simulink model "Droop_GC"  (Simulink 9.1)
settings: Solver=ode4  StartTime=0.0  StopTime=2.6  FixedStep=1e-6  RelTol=1e-3  EnableMultiTasking=on
InitFcn:
  | %% Circuit parameters
  | % LC filter
  | Lf_1 = 1.35e-3;
  | Rf_1 = 0.1;
  | Cf_1 = 50e-6;
  | 
  | Lf_2 = 1.35e-3;
  | Rf_2 = 0.1;
  | Cf_2 = 50e-6;
  | 
  | Lf_3 = 1.35e-3;
  | Rf_3 = 0.1;
  | Cf_3 = 50e-6;
  | 
  | % transmission line(grid coupling impedance)
  | L_1 = 0.35e-3;
  | R_1 = 0.03;
  | 
  | L_2 = 0.35e-3;
  | R_2 = 0.03;
  | 
  | L_3 = 0.35e-3;
  | R_3 = 0.03;
  | 
  | % Network
  | % active power loop
  | fn = 50;
  | wn = 2*pi*fn;
  | 
  | R_line_1 = 0.23;
  | L_line_1 = 0.1 / wn;
  | 
  | R_line_2 = 0.35;
  | L_line_2 = 0.58 / wn;
  | 
  | 
  | %% Control parameters
  | % power measurement LPF
  | wc = 31.41;
  | 
  | % Power droop
  | mp_1 = mp;
  | mp_2 = mp;
  | mp_3 = mp;
  | 
  | nq_1 = nq;
  | nq_2 = nq;
  | nq_3 = nq;
  | 
  | J1 = 0.1;
  | J2 = 0.1;
  | J3 = 0.1;
  | 
  | Pref_1 = Pref;
  | Pref_2 = Pref;
  | Pref_3 = Pref;
  | 
  | % outer voltage loop
  | Kpv_1 = 0.05;
  | Kiv_1 = 390;
  | F_1 = 1;
  | 
  | Kpv_2 = 0.05;
  | Kiv_2 = 390;
  | F_2 = 1;
  | 
  | Kpv_3 = 0.05;
  | Kiv_3 = 390;
  | F_3 = 1;
  | 
  | % inner current control loop
  | Kpc_1 = 10.5;
  | Kic_1 = 16e3;
  | 
  | Kpc_2 = 10.5;
  | Kic_2 = 16e3;
  | 
  | Kpc_3 = 10.5;
  | Kic_3 = 16e3;
  | % ?? reference voltage
  | 
  | V_phase_rms = 220;
  | V_line_rms = V_phase_rms * sqrt(3);
  | 
  | % Load
  | R_load_1 = R1;
  | L_load_1 = 10e-9;
  | 
  | R_load_2 = R3;
  | L_load_2 = 10e-9;
  | 
  | 
  | % Pre Synchronisation for Con 1
  | t_grid_breaker = 0.6;
  | t_preSyn_start = 0.01;
  | t_preSyn_end = t_grid_breaker;
  | 
  | % Pre Synchronisation for Con 2
  | t_grid_breaker_2 = 1.2;
  | t_preSyn_start_2 = 0.61;
  | t_preSyn_end_2 = t_grid_breaker_2;
  | 
  | 
  | % Pre Synchronisation for Con 3
  | t_grid_breaker_3 = 1.8;
  | t_preSyn_start_3 = 1.21;
  | t_preSyn_end_3 = t_grid_breaker_3;
  | 
  | % PLL
  | Vg = V_phase_rms * sqrt(2);
  | % Disturbance Rejection
  | wd = 2*pi*100;                      % Definition of 1st Harmonic Band
  | att_lim = 20*log10((5e-3)/108);      % Defintion of Damping here: 5e-3 maximum tolerance and 108 V Type E negative sequence Voltage
  | 
  | a = 2.4;                            % corresponds xi = 0.7
  | 
  | wc_lim = wd*sqrt(Vg)/sqrt(a)*10^(att_lim/40);    % calculation of bandwidth
  | 
  | Kp_pll = wc_lim;
  | wf_pll = a*wc_lim;      %1/sqrt(2)*w0;
  | T_L = 1/wf_pll;
  | Ki_pll = Kp_pll*wc_lim/a;
  | Ti_pll = Kp_pll/Ki_pll;
  | 
  | %% Pre synchronization PI parameters? G_cl =(Kp_syn*s + Ki_syn) / (s^2 + Kp_syn*s + Ki_syn)
  | % ? = 0.707? ts = ??
  | ts_syn = 0.5;
  | zeta_syn = 0.707;
  | wn_syn = 4.5 / (ts_syn * zeta_syn);
  | 
  | Ki_syn = wn_syn * wn_syn;
  | Kp_syn = 2 * zeta_syn * wn_syn;
  | 
  | 
  | Udc = 800;
  | fs = 8000;
values from neighbouring files (symbols this model uses):
  mp = 9.4e-5    (= 9.4e-05)    [model_coefficient.m]
  nq = 1.3e-3    (= 0.0013)    [model_coefficient.m]
  Pref = 10000    [model_coefficient.m]
  R1 = 25    [model_coefficient.m]
  R3 = 20    [model_coefficient.m]
libraries: powerlib x53, powerlib_meascontrol x25
(part 1 of 2)
Description:
  | Model of a simple control system for use iin training.
settings Model: ARTEMISmethode_block_infos=$$__separator__$$Droop_GC/ARTEMIS Guide$$__separator__$$  Creator=Paul Baracos  LastModifiedBy=10135
settings DataIOCC: LimitDataPoints=on  SignalLoggingSaveFormat=ModelDataLogs  SaveOutput=off  SaveTime=off  ReturnWorkspaceOutputs=on  SignalLoggingName=sigsOut  LoggingIntervals=[2.599, 2.6]
settings OptimizationCC: BlockReduction=off  BooleanDataType=off  OptimizeBlockIOStorage=off  BufferReuse=off  GlobalBufferReuse=off  ExpressionFolding=off  LocalBlockOutputs=off  InitFltsAndDblsToZero=on  OptimizeDataStoreBuffers=off  BusAssignmentInplaceUpdate=off
settings DebuggingCC: SaveWithParameterizedLinksMsg=none  SignalResolutionControl=TryResolveAllWithWarning  MultiTaskDSMMsg=warning  MultiTaskCondExecSysMsg=none  FcnCallInpInsideContextMsg=warning
settings HardwareCC: TargetUnknown=on
settings GRTTargetCC: TargetFcnLib=ansi_tfl_tmw.mat  GeneratePreprocessorConditionals=Disable all
settings SimscapeCC: SimscapeNormalizeSystem=off  SimscapeLogType=local  SimscapeLogLimitData=off

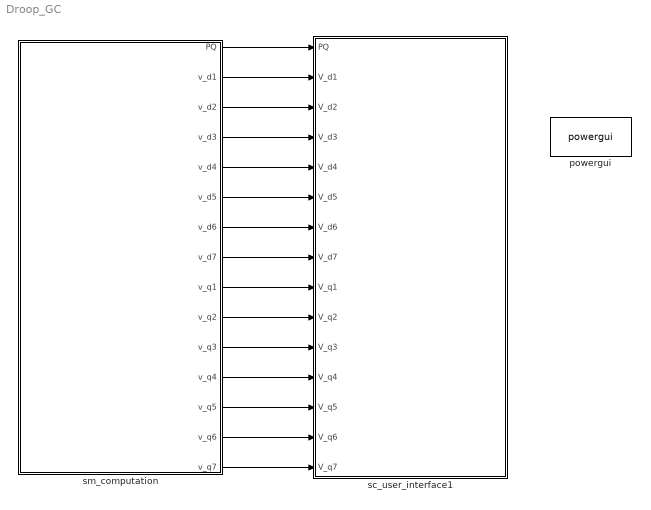
== system Droop_GC ==
  powergui : powerlib/powergui  Priority=1  SimulationMode=Discrete  SampleTime=1e-6  frequency=60  Iterations=50  frequencyindice=0  Pbase=100e6  ErrMax=1e-4  UnitsV=kV  UnitsW=MW  buscounter=0  FunctionMessages=off  echomessages=off  EnableUseOfTLC=off  CurrentSourceSwitches=off  DisableSnubberDevices=off  DisableRonSwitches=off  DisableVfSwitches=off  DisplayEquations=off  SolverType=Tustin/Backward Euler (TBE)  Interpol=off  ExternalGateDelay=off  methode=off  Ts=100  x0status=blocks  SPID=off  SwTol=0  HookPort=off  RestoreLinks=warning  ResistiveCurrentMeasurement=off  Frange=[0:2:500]  Ylog=off  Xlog=on  ShowGrid=off  save=off  variable=ZData  structure=0  ZoomFFT=off  StartTime=0.0  cycles=1  DisplayStyle=1  fundamental=60  FreqAxis=off  MaxFrequency=1000  frequencyindicesteady=1  RmsSteady=1  display=off
  sc_user_interface1 : Subsystem
  sm_computation : Subsystem
  wires:
  sm_computation/1(PQ) -> sc_user_interface1/1(PQ)
  sm_computation/2(v_d1) -> sc_user_interface1/2(V_d1)
  sm_computation/3(v_d2) -> sc_user_interface1/3(V_d2)
  sm_computation/4(v_d3) -> sc_user_interface1/4(V_d3)
  sm_computation/5(v_d4) -> sc_user_interface1/5(V_d4)
  sm_computation/6(v_d5) -> sc_user_interface1/6(V_d5)
  sm_computation/7(v_d6) -> sc_user_interface1/7(V_d6)
  sm_computation/8(v_d7) -> sc_user_interface1/8(V_d7)
  sm_computation/9(v_q1) -> sc_user_interface1/9(V_q1)
  sm_computation/10(v_q2) -> sc_user_interface1/10(V_q2)
  sm_computation/11(v_q3) -> sc_user_interface1/11(V_q3)
  sm_computation/12(v_q4) -> sc_user_interface1/12(V_q4)
  sm_computation/13(v_q5) -> sc_user_interface1/13(V_q5)
  sm_computation/14(v_q6) -> sc_user_interface1/14(V_q6)
  sm_computation/15(v_q7) -> sc_user_interface1/15(V_q7)

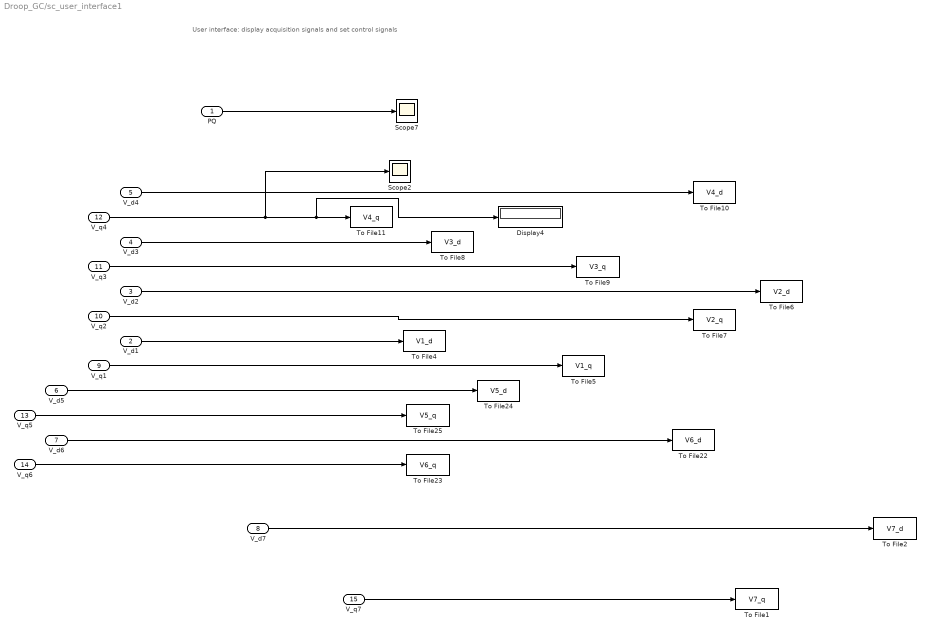
== system Droop_GC/sc_user_interface1 ==
  note: User interface: display acquisition signals and set control signals
  PQ : Inport
  V_d1 : Inport  Port=2
  V_d2 : Inport  Port=3
  V_d3 : Inport  Port=4
  V_d4 : Inport  Port=5
  V_d5 : Inport  Port=6
  V_d6 : Inport  Port=7
  V_d7 : Inport  Port=8
  V_q1 : Inport  Port=9
  V_q2 : Inport  Port=10
  V_q3 : Inport  Port=11
  V_q4 : Inport  Port=12
  V_q5 : Inport  Port=13
  V_q6 : Inport  Port=14
  V_q7 : Inport  Port=15
  Display4 : Display
  Scope2 : Scope
      settings: Tag=op_tm_save_it
  Scope7 : Scope
      settings: Tag=op_tm_save_it
  To File1 : ToFile  Filename=V7_q  SaveFormat=Timeseries
  To File10 : ToFile  Filename=V4_d  SaveFormat=Timeseries
  To File11 : ToFile  Filename=V4_q  SaveFormat=Timeseries
  To File2 : ToFile  Filename=V7_d  SaveFormat=Timeseries
  To File22 : ToFile  Filename=V6_d  SaveFormat=Timeseries
  To File23 : ToFile  Filename=V6_q  SaveFormat=Timeseries
  To File24 : ToFile  Filename=V5_d  SaveFormat=Timeseries
  To File25 : ToFile  Filename=V5_q  SaveFormat=Timeseries
  To File4 : ToFile  Filename=V1_d  SaveFormat=Timeseries
  To File5 : ToFile  Filename=V1_q  SaveFormat=Timeseries
  To File6 : ToFile  Filename=V2_d  SaveFormat=Timeseries
  To File7 : ToFile  Filename=V2_q  SaveFormat=Timeseries
  To File8 : ToFile  Filename=V3_d  SaveFormat=Timeseries
  To File9 : ToFile  Filename=V3_q  SaveFormat=Timeseries
  wires:
  PQ/1 -> Scope7/1
  V_d6/1 -> To File22/1
  V_d2/1 -> To File6/1
  V_q3/1 -> To File9/1
  V_q2/1 -> To File7/1
  V_q5/1 -> To File25/1
  V_d5/1 -> To File24/1
  V_d3/1 -> To File8/1
  V_q6/1 -> To File23/1
  V_d1/1 -> To File4/1
  V_q1/1 -> To File5/1
  V_q4/1 -> Scope2/1, Display4/1, To File11/1
  V_d4/1 -> To File10/1
  V_q7/1 -> To File1/1
  V_d7/1 -> To File2/1

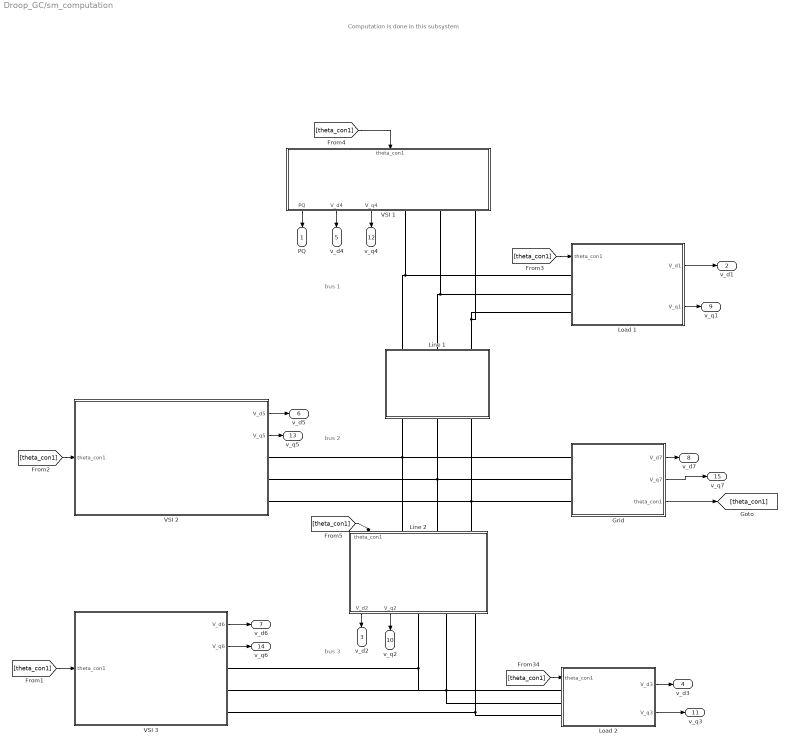
== system Droop_GC/sm_computation ==
  note: Computation is done in this subsystem
  note: bus 1
  note: bus 3
  note: bus 2
  Grid : Subsystem
  Line 1 : Subsystem
  Line 2 : Subsystem
  Load 1 : Subsystem
  Load 2 : Subsystem
  VSI 1 : Subsystem
  VSI 2 : Subsystem
  VSI 3 : Subsystem
  PQ : Outport
  v_d1 : Outport  Port=2
  v_d2 : Outport  Port=3
  v_d3 : Outport  Port=4
  v_d4 : Outport  Port=5
  v_d5 : Outport  Port=6
  v_d6 : Outport  Port=7
  v_d7 : Outport  Port=8
  v_q1 : Outport  Port=9
  v_q2 : Outport  Port=10
  v_q3 : Outport  Port=11
  v_q4 : Outport  Port=12
  v_q5 : Outport  Port=13
  v_q6 : Outport  Port=14
  v_q7 : Outport  Port=15
  wires:
  Grid/3(theta_con1) -> [theta_con1]
  [theta_con1] -> Load 2/1("theta_con1 ")
  [theta_con1] -> VSI 3/1("theta_con1 ")
  [theta_con1] -> VSI 2/1("theta_con1 ")
  [theta_con1] -> Load 1/1("theta_con1 ")
  [theta_con1] -> VSI 1/1("theta_con1 ")
  VSI 1/1(PQ) -> PQ/1
  Load 1/1(V_d1) -> v_d1/1
  Line 2/1(V_d2) -> v_d2/1
  Load 2/1(V_d3) -> v_d3/1
  VSI 1/2(V_d4) -> v_d4/1
  VSI 2/1(V_d5) -> v_d5/1
  VSI 3/1(V_d6) -> v_d6/1
  Grid/1(V_d7) -> v_d7/1
  Load 1/2(V_q1) -> v_q1/1
  Line 2/2(V_q2) -> v_q2/1
  Load 2/2(V_q3) -> v_q3/1
  VSI 1/3(V_q4) -> v_q4/1
  VSI 2/2(V_q5) -> v_q5/1
  VSI 3/2(V_q6) -> v_q6/1
  Grid/2(V_q7) -> v_q7/1
  [theta_con1] -> Line 2/1("theta_con1 ")
  connections:
  Load 2/LConn1 -- VSI 3/RConn1 -- Line 2/RConn1
  VSI 1/RConn1 -- Load 1/LConn1 -- Line 1/LConn1
  VSI 1/RConn3 -- Line 1/LConn3 -- Load 1/LConn3
  Grid/LConn1 -- Line 2/LConn1 -- VSI 2/RConn1 -- Line 1/RConn1
  Grid/LConn3 -- Line 2/LConn3 -- VSI 2/RConn3 -- Line 1/RConn3
  Load 2/LConn2 -- VSI 3/RConn2 -- Line 2/RConn2
  VSI 1/RConn2 -- Line 1/LConn2 -- Load 1/LConn2
  Grid/LConn2 -- Line 2/LConn2 -- VSI 2/RConn2 -- Line 1/RConn2
  Load 2/LConn3 -- VSI 3/RConn3 -- Line 2/RConn3

== system Droop_GC/sm_computation/Grid ==
  Constant1 : Constant  Value=2*pi/3
  Constant3 : Constant  Value=wn
  Demux : Demux  Outputs=3
  Demux1 : Demux  Outputs=3
  Gain : Gain  Gain=Vg
  Integrator3 : Integrator
  Mux : Mux  Inputs=3
  Sum : Sum  Inputs=|+-
  Sum1 : Sum  Inputs=++|
  Terminator2 : Terminator
  Three-Phase Series RLC Branch : powerlib/Elements/Three-Phase Series RLC Branch  LConnTagsString=A|B|C  RConnTagsString=A|B|C  BranchType=RL  Resistance=R_line_1  Inductance=L_line_1  Capacitance=1e-6  Measurements=None
  Three-Phase V-I Measurement : powerlib/Measurements/Three-Phase V-I Measurement  VoltageMeasurement=phase-to-ground  SetLabelV=off  LabelV=Vabc  Vpu=off  VpuLL=off  CurrentMeasurement=no  SetLabelI=off  LabelI=Iabc  Ipu=off  Pbase=100e6  Vbase=500e3  OutputType=Complex  PhasorSimulation=off  PSBequivalent=0
  Trigonometric Function : Trigonometry  Operator=cos
  Trigonometric Function1 : Trigonometry  Operator=cos
  Trigonometric Function2 : Trigonometry  Operator=cos
  abc to dq0 : powerlib_meascontrol/Transformations/abc to dq0  Alignment=Aligned with phase A axis
  u1 : powerlib/Electrical Sources/Controlled Voltage Source  Initialize=off  Source_Type=AC  Amplitude=0  Phase=0  Frequency=50  Measurements=None
  u2 : powerlib/Electrical Sources/Controlled Voltage Source  Initialize=off  Source_Type=AC  Amplitude=0  Phase=0  Frequency=50  Measurements=None
  u3 : powerlib/Electrical Sources/Controlled Voltage Source  Initialize=off  Source_Type=AC  Amplitude=0  Phase=0  Frequency=50  Measurements=None
  A : PMIOPort  Side=Left
  B : PMIOPort  Port=2  Side=Left
  C : PMIOPort  Port=3  Side=Left
  V_d7 : Outport
  V_q7 : Outport  Port=2
  theta_con1 : Outport  Port=3
  tag scope: theta_con1=global
  wires:
  Constant3/1 -> Integrator3/1
  Integrator3/1 -> Trigonometric Function/1, Sum1/2, Sum/1, theta_con1/1, [theta_con1]
  Demux/2 -> u2/1
  Demux/1 -> u1/1
  Demux/3 -> u3/1
  Constant1/1 -> Sum1/1, Sum/2
  Sum1/1 -> Trigonometric Function2/1
  Sum/1 -> Trigonometric Function1/1
  Trigonometric Function/1 -> Mux/1
  Trigonometric Function2/1 -> Mux/3
  Trigonometric Function1/1 -> Mux/2
  Mux/1 -> Gain/1
  Gain/1 -> Demux/1
  Demux1/2 -> V_q7/1
  abc to dq0/1 -> Demux1/1
  Three-Phase V-I Measurement/1 -> abc to dq0/1
  [theta_con1] -> abc to dq0/2
  Demux1/3 -> Terminator2/1
  Demux1/1 -> V_d7/1
  connections:
  Three-Phase V-I Measurement/RConn2 -- u2/RConn1
  Three-Phase V-I Measurement/RConn1 -- u1/RConn1
  Three-Phase V-I Measurement/RConn3 -- u3/RConn1
  Three-Phase Series RLC Branch/RConn1 -- Three-Phase V-I Measurement/LConn1
  Three-Phase Series RLC Branch/RConn2 -- Three-Phase V-I Measurement/LConn2
  Three-Phase Series RLC Branch/RConn3 -- Three-Phase V-I Measurement/LConn3
  Three-Phase Series RLC Branch/LConn1 -- A/RConn1
  Three-Phase Series RLC Branch/LConn2 -- B/RConn1
  Three-Phase Series RLC Branch/LConn3 -- C/RConn1
  u1/LConn1 -- u3/LConn1 -- u2/LConn1

== system Droop_GC/sm_computation/Line 1 ==
  Three-Phase Series RLC Branch : powerlib/Elements/Three-Phase Series RLC Branch  LConnTagsString=A|B|C  RConnTagsString=A|B|C  BranchType=RL  Resistance=R_line_1  Inductance=L_line_1  Capacitance=1e-6  Measurements=None
  Three-Phase V-I Measurement : powerlib/Measurements/Three-Phase V-I Measurement  VoltageMeasurement=phase-to-ground  SetLabelV=off  LabelV=Vabc  Vpu=off  VpuLL=off  CurrentMeasurement=yes  SetLabelI=off  LabelI=Iabc  Ipu=off  Pbase=100e6  Vbase=500e3  OutputType=Complex  PhasorSimulation=off  PSBequivalent=0
  a : PMIOPort  Side=Right
  b : PMIOPort  Port=2  Side=Right
  c : PMIOPort  Port=3  Side=Right
  A1 : PMIOPort  Port=4  Side=Left
  B1 : PMIOPort  Port=5  Side=Left
  C1 : PMIOPort  Port=6  Side=Left
  tag scope: I_line_1_abc=global, V_b_1_abc=global
  wires:
  Three-Phase V-I Measurement/1 -> [V_b_1_abc]
  Three-Phase V-I Measurement/2 -> [I_line_1_abc]
  connections:
  Three-Phase Series RLC Branch/RConn1 -- a/RConn1
  Three-Phase Series RLC Branch/RConn2 -- b/RConn1
  Three-Phase Series RLC Branch/RConn3 -- c/RConn1
  Three-Phase Series RLC Branch/LConn2 -- Three-Phase V-I Measurement/RConn2
  C1/RConn1 -- Three-Phase V-I Measurement/LConn3
  B1/RConn1 -- Three-Phase V-I Measurement/LConn2
  Three-Phase Series RLC Branch/LConn3 -- Three-Phase V-I Measurement/RConn3
  A1/RConn1 -- Three-Phase V-I Measurement/LConn1
  Three-Phase Series RLC Branch/LConn1 -- Three-Phase V-I Measurement/RConn1

== system Droop_GC/sm_computation/Line 2 ==
  "theta_con1 " : Inport
  Demux : Demux  Outputs=3
  Terminator2 : Terminator
  Three-Phase Series RLC Branch : powerlib/Elements/Three-Phase Series RLC Branch  LConnTagsString=A|B|C  RConnTagsString=A|B|C  BranchType=RL  Resistance=R_line_2  Inductance=L_line_2  Capacitance=1e-6  Measurements=None
  Three-Phase V-I Measurement : powerlib/Measurements/Three-Phase V-I Measurement  VoltageMeasurement=phase-to-ground  SetLabelV=off  LabelV=Vabc  Vpu=off  VpuLL=off  CurrentMeasurement=no  SetLabelI=off  LabelI=Iabc  Ipu=off  Pbase=100e6  Vbase=500e3  OutputType=Complex  PhasorSimulation=off  PSBequivalent=0
  Three-Phase V-I Measurement1 : powerlib/Measurements/Three-Phase V-I Measurement  VoltageMeasurement=no  SetLabelV=off  LabelV=Vabc  Vpu=off  VpuLL=off  CurrentMeasurement=no  SetLabelI=off  LabelI=Iabc  Ipu=off  Pbase=100e6  Vbase=500e3  OutputType=Complex  PhasorSimulation=off  PSBequivalent=0
  abc to dq0 : powerlib_meascontrol/Transformations/abc to dq0  Alignment=Aligned with phase A axis
  a : PMIOPort  Side=Right
  b : PMIOPort  Port=2  Side=Right
  c : PMIOPort  Port=3  Side=Right
  A1 : PMIOPort  Port=4  Side=Left
  B1 : PMIOPort  Port=5  Side=Left
  C1 : PMIOPort  Port=6  Side=Left
  V_d2 : Outport
  V_q2 : Outport  Port=2
  wires:
  Demux/3 -> Terminator2/1
  Demux/2 -> V_q2/1
  Three-Phase V-I Measurement/1 -> abc to dq0/1
  "theta_con1 "/1 -> abc to dq0/2
  abc to dq0/1 -> Demux/1
  Demux/1 -> V_d2/1
  connections:
  B1/RConn1 -- Three-Phase V-I Measurement/LConn2
  Three-Phase Series RLC Branch/LConn2 -- Three-Phase V-I Measurement/RConn2
  Three-Phase V-I Measurement/RConn1 -- Three-Phase Series RLC Branch/LConn1
  Three-Phase V-I Measurement/RConn3 -- Three-Phase Series RLC Branch/LConn3
  A1/RConn1 -- Three-Phase V-I Measurement/LConn1
  C1/RConn1 -- Three-Phase V-I Measurement/LConn3
  Three-Phase Series RLC Branch/RConn1 -- Three-Phase V-I Measurement1/LConn1
  Three-Phase Series RLC Branch/RConn2 -- Three-Phase V-I Measurement1/LConn2
  Three-Phase Series RLC Branch/RConn3 -- Three-Phase V-I Measurement1/LConn3
  c/RConn1 -- Three-Phase V-I Measurement1/RConn3
  b/RConn1 -- Three-Phase V-I Measurement1/RConn2
  a/RConn1 -- Three-Phase V-I Measurement1/RConn1

== system Droop_GC/sm_computation/Load 1 ==
  "theta_con1 " : Inport
  Demux : Demux  Outputs=3
  Ground2 : powerlib/Elements/Ground  LConnTagsString=a
  Terminator2 : Terminator
  Three-Phase Series RLC Branch : powerlib/Elements/Three-Phase Series RLC Branch  LConnTagsString=A|B|C  RConnTagsString=A|B|C  BranchType=RL  Resistance=R_load_1  Inductance=L_load_1  Capacitance=1e-6  Measurements=None
  Three-Phase V-I Measurement : powerlib/Measurements/Three-Phase V-I Measurement  VoltageMeasurement=phase-to-ground  SetLabelV=off  LabelV=Vabc  Vpu=off  VpuLL=off  CurrentMeasurement=no  SetLabelI=off  LabelI=Iabc  Ipu=off  Pbase=100e6  Vbase=500e3  OutputType=Complex  PhasorSimulation=off  PSBequivalent=0
  abc to dq0 : powerlib_meascontrol/Transformations/abc to dq0  Alignment=Aligned with phase A axis
  A : PMIOPort  Side=Left
  B : PMIOPort  Port=2  Side=Left
  C : PMIOPort  Port=3  Side=Left
  V_d1 : Outport
  V_q1 : Outport  Port=2
  wires:
  abc to dq0/1 -> Demux/1
  Three-Phase V-I Measurement/1 -> abc to dq0/1
  Demux/2 -> V_q1/1
  Demux/3 -> Terminator2/1
  Demux/1 -> V_d1/1
  "theta_con1 "/1 -> abc to dq0/2
  connections:
  Ground2/LConn1 -- Three-Phase Series RLC Branch/RConn3 -- Three-Phase Series RLC Branch/RConn1 -- Three-Phase Series RLC Branch/RConn2
  Three-Phase V-I Measurement/RConn2 -- Three-Phase Series RLC Branch/LConn2
  Three-Phase V-I Measurement/RConn1 -- Three-Phase Series RLC Branch/LConn1
  Three-Phase V-I Measurement/RConn3 -- Three-Phase Series RLC Branch/LConn3
  A/RConn1 -- Three-Phase V-I Measurement/LConn1
  B/RConn1 -- Three-Phase V-I Measurement/LConn2
  C/RConn1 -- Three-Phase V-I Measurement/LConn3

== system Droop_GC/sm_computation/Load 2 ==
  "theta_con1 " : Inport
  Demux : Demux  Outputs=3
  Ground2 : powerlib/Elements/Ground  LConnTagsString=a
  Terminator2 : Terminator
  Three-Phase Series RLC Branch : powerlib/Elements/Three-Phase Series RLC Branch  LConnTagsString=A|B|C  RConnTagsString=A|B|C  BranchType=RL  Resistance=R_load_2  Inductance=L_load_2  Capacitance=1e-6  Measurements=None
  Three-Phase V-I Measurement : powerlib/Measurements/Three-Phase V-I Measurement  VoltageMeasurement=phase-to-ground  SetLabelV=off  LabelV=Vabc  Vpu=off  VpuLL=off  CurrentMeasurement=no  SetLabelI=off  LabelI=Iabc  Ipu=off  Pbase=100e6  Vbase=500e3  OutputType=Complex  PhasorSimulation=off  PSBequivalent=0
  abc to dq0 : powerlib_meascontrol/Transformations/abc to dq0  Alignment=Aligned with phase A axis
  A : PMIOPort  Side=Left
  B : PMIOPort  Port=2  Side=Left
  C : PMIOPort  Port=3  Side=Left
  V_d3 : Outport
  V_q3 : Outport  Port=2
  wires:
  Demux/2 -> V_q3/1
  abc to dq0/1 -> Demux/1
  Three-Phase V-I Measurement/1 -> abc to dq0/1
  "theta_con1 "/1 -> abc to dq0/2
  Demux/3 -> Terminator2/1
  Demux/1 -> V_d3/1
  connections:
  Three-Phase Series RLC Branch/RConn1 -- Ground2/LConn1 -- Three-Phase Series RLC Branch/RConn3 -- Three-Phase Series RLC Branch/RConn2
  Three-Phase Series RLC Branch/LConn2 -- Three-Phase V-I Measurement/RConn2
  C/RConn1 -- Three-Phase V-I Measurement/LConn3
  B/RConn1 -- Three-Phase V-I Measurement/LConn2
  Three-Phase V-I Measurement/RConn3 -- Three-Phase Series RLC Branch/LConn3
  A/RConn1 -- Three-Phase V-I Measurement/LConn1
  Three-Phase V-I Measurement/RConn1 -- Three-Phase Series RLC Branch/LConn1

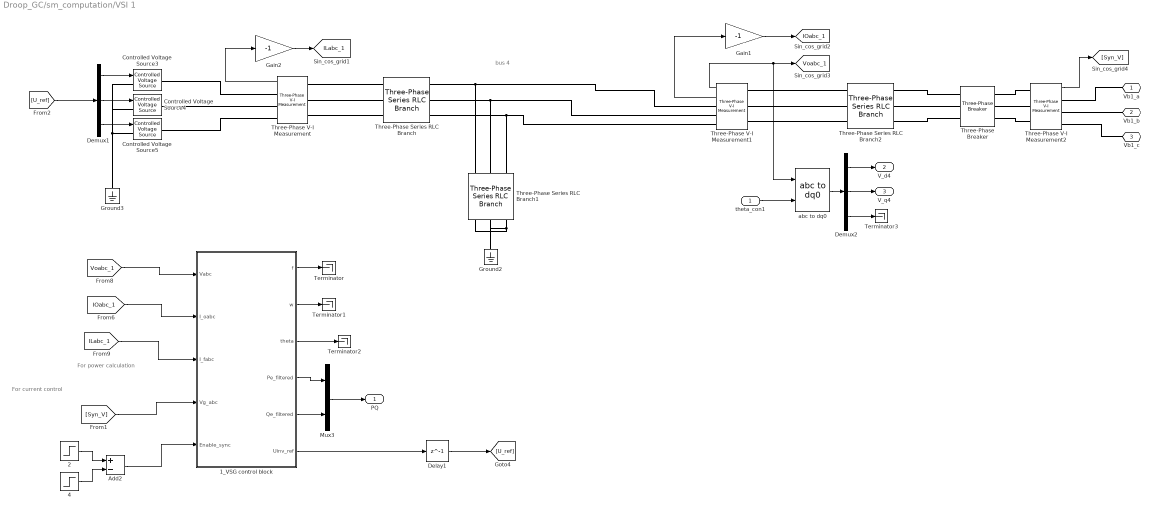
== system Droop_GC/sm_computation/VSI 1 ==
  note: For power calculation
  note: For current control
  note: bus 4
  "theta_con1 " : Inport
  " 2" : Step  Time=t_preSyn_start  SampleTime=0
  " 4" : Step  Time=t_preSyn_end  SampleTime=0
  1_VSG control block : Subsystem
  Add2 : Sum  Inputs=+-
  Controlled Voltage Source3 : powerlib/Electrical Sources/Controlled Voltage Source  Initialize=on  Source_Type=AC  Amplitude=0  Phase=0  Frequency=0  Measurements=None
  Controlled Voltage Source4 : powerlib/Electrical Sources/Controlled Voltage Source  Initialize=on  Source_Type=AC  Amplitude=0  Phase=0  Frequency=0  Measurements=None
  Controlled Voltage Source5 : powerlib/Electrical Sources/Controlled Voltage Source  Initialize=on  Source_Type=AC  Amplitude=0  Phase=0  Frequency=0  Measurements=None
  Delay1 : Delay  DelayLength=1  InitialCondition=0
  Demux1 : Demux  Outputs=3
  Demux2 : Demux  Outputs=3
  Gain1 : Gain  Gain=-1
  Gain2 : Gain  Gain=-1
  Ground2 : powerlib/Elements/Ground  LConnTagsString=a
  Ground3 : powerlib/Elements/Ground  LConnTagsString=a
  Mux3 : Mux  Inputs=2
  Terminator{,1..3} (4 alike) : Terminator
  Three-Phase Series RLC Branch : powerlib/Elements/Three-Phase Series RLC Branch  LConnTagsString=A|B|C  RConnTagsString=A|B|C  BranchType=RL  Resistance=Rf_1  Inductance=Lf_1  Capacitance=1e-6  Measurements=None
  Three-Phase Series RLC Branch1 : powerlib/Elements/Three-Phase Series RLC Branch  LConnTagsString=A|B|C  RConnTagsString=A|B|C  BranchType=C  Resistance=Rf_1  Inductance=0.1e-3  Capacitance=Cf_1  Measurements=None
  Three-Phase Series RLC Branch2 : powerlib/Elements/Three-Phase Series RLC Branch  LConnTagsString=A|B|C  RConnTagsString=A|B|C  BranchType=RL  Resistance=R_1  Inductance=L_1  Capacitance=1e-6  Measurements=None
  Three-Phase V-I Measurement : powerlib/Measurements/Three-Phase V-I Measurement  VoltageMeasurement=no  SetLabelV=off  LabelV=Vabc  Vpu=off  VpuLL=off  CurrentMeasurement=yes  SetLabelI=off  LabelI=Iabc  Ipu=off  Pbase=100e6  Vbase=500e3  OutputType=Complex  PhasorSimulation=off  PSBequivalent=0
  Three-Phase V-I Measurement1 : powerlib/Measurements/Three-Phase V-I Measurement  VoltageMeasurement=phase-to-ground  SetLabelV=off  LabelV=Vabc  Vpu=off  VpuLL=off  CurrentMeasurement=yes  SetLabelI=off  LabelI=Iabc  Ipu=off  Pbase=100e6  Vbase=500e3  OutputType=Complex  PhasorSimulation=off  PSBequivalent=0
  Three-Phase V-I Measurement2 : powerlib/Measurements/Three-Phase V-I Measurement  VoltageMeasurement=phase-to-ground  SetLabelV=off  LabelV=Vabc  Vpu=off  VpuLL=off  CurrentMeasurement=no  SetLabelI=off  LabelI=Iabc  Ipu=off  Pbase=100e6  Vbase=500e3  OutputType=Complex  PhasorSimulation=off  PSBequivalent=0
  Three-Phase Breaker : powerlib/Elements/Three-Phase Breaker  InitialState=open  SwitchA=on  SwitchB=on  SwitchC=on  SwitchTimes="[t_grid_breaker  20]"  External=off  BreakerResistance=0.00001  SnubberResistance=1e8  SnubberCapacitance=inf  Measurements=None
  abc to dq0 : powerlib_meascontrol/Transformations/abc to dq0  Alignment=Aligned with phase A axis
  Vb1_a : PMIOPort  Side=Right
  Vb1_b : PMIOPort  Port=2  Side=Right
  Vb1_c : PMIOPort  Port=3  Side=Right
  PQ : Outport
  V_d4 : Outport  Port=2
  V_q4 : Outport  Port=3
  tag scope: ILabc_1=global, IOabc_1=global, Voabc_1=global
  wires:
  [ILabc_1] -> 1_VSG control block/3(I_fabc)
  [Voabc_1] -> 1_VSG control block/1(Vabc)
  [IOabc_1] -> 1_VSG control block/2(I_oabc)
  Mux3/1 -> PQ/1
  1_VSG control block/4(Pe_filtered) -> Mux3/1
  1_VSG control block/5(Qe_filtered) -> Mux3/2
  1_VSG control block/2(w) -> Terminator1/1
  1_VSG control block/1(f) -> Terminator/1
  Three-Phase V-I Measurement2/1 -> [Syn_V]
  [Syn_V] -> 1_VSG control block/4(Vg_abc)
  " 2"/1 -> Add2/1
  " 4"/1 -> Add2/2
  Add2/1 -> 1_VSG control block/5(Enable_sync)
  1_VSG control block/3(theta) -> Terminator2/1
  Three-Phase V-I Measurement/1 -> Gain2/1
  Gain1/1 -> [IOabc_1]
  Three-Phase V-I Measurement1/2 -> Gain1/1
  Three-Phase V-I Measurement1/1 -> abc to dq0/1, [Voabc_1]
  Gain2/1 -> [ILabc_1]
  1_VSG control block/6(Uinv_ref) -> Delay1/1
  Delay1/1 -> [U_ref]
  [U_ref] -> Demux1/1
  Demux1/3 -> Controlled Voltage Source5/1
  Demux1/1 -> Controlled Voltage Source3/1
  Demux1/2 -> Controlled Voltage Source4/1
  Demux2/1 -> V_d4/1
  Demux2/2 -> V_q4/1
  Demux2/3 -> Terminator3/1
  abc to dq0/1 -> Demux2/1
  "theta_con1 "/1 -> abc to dq0/2
  connections:
  Three-Phase Series RLC Branch2/RConn2 -- Three-Phase Breaker/LConn2
  Three-Phase Series RLC Branch2/RConn1 -- Three-Phase Breaker/LConn1
  Three-Phase Series RLC Branch2/RConn3 -- Three-Phase Breaker/LConn3
  Three-Phase V-I Measurement2/LConn2 -- Three-Phase Breaker/RConn2
  Three-Phase Breaker/RConn1 -- Three-Phase V-I Measurement2/LConn1
  Three-Phase Breaker/RConn3 -- Three-Phase V-I Measurement2/LConn3
  Three-Phase V-I Measurement2/RConn1 -- Vb1_a/RConn1
  Three-Phase V-I Measurement2/RConn2 -- Vb1_b/RConn1
  Three-Phase V-I Measurement2/RConn3 -- Vb1_c/RConn1
  Three-Phase Series RLC Branch1/RConn3 -- Ground2/LConn1 -- Three-Phase Series RLC Branch1/RConn1 -- Three-Phase Series RLC Branch1/RConn2
  Three-Phase Series RLC Branch/RConn3 -- Three-Phase Series RLC Branch1/LConn3 -- Three-Phase V-I Measurement1/RConn3
  Three-Phase Series RLC Branch/RConn2 -- Three-Phase Series RLC Branch1/LConn2 -- Three-Phase V-I Measurement1/RConn2
  Three-Phase V-I Measurement1/LConn3 -- Three-Phase Series RLC Branch2/LConn3
  Three-Phase Series RLC Branch/RConn1 -- Three-Phase Series RLC Branch1/LConn1 -- Three-Phase V-I Measurement1/RConn1
  Three-Phase V-I Measurement1/LConn1 -- Three-Phase Series RLC Branch2/LConn1
  Three-Phase V-I Measurement1/LConn2 -- Three-Phase Series RLC Branch2/LConn2
  Three-Phase V-I Measurement/LConn3 -- Three-Phase Series RLC Branch/LConn3
  Three-Phase V-I Measurement/LConn2 -- Three-Phase Series RLC Branch/LConn2
  Three-Phase V-I Measurement/LConn1 -- Three-Phase Series RLC Branch/LConn1
  Controlled Voltage Source5/LConn1 -- Controlled Voltage Source4/LConn1 -- Controlled Voltage Source3/LConn1 -- Ground3/LConn1
  Three-Phase V-I Measurement/RConn2 -- Controlled Voltage Source4/RConn1
  Three-Phase V-I Measurement/RConn3 -- Controlled Voltage Source5/RConn1
  Three-Phase V-I Measurement/RConn1 -- Controlled Voltage Source3/RConn1

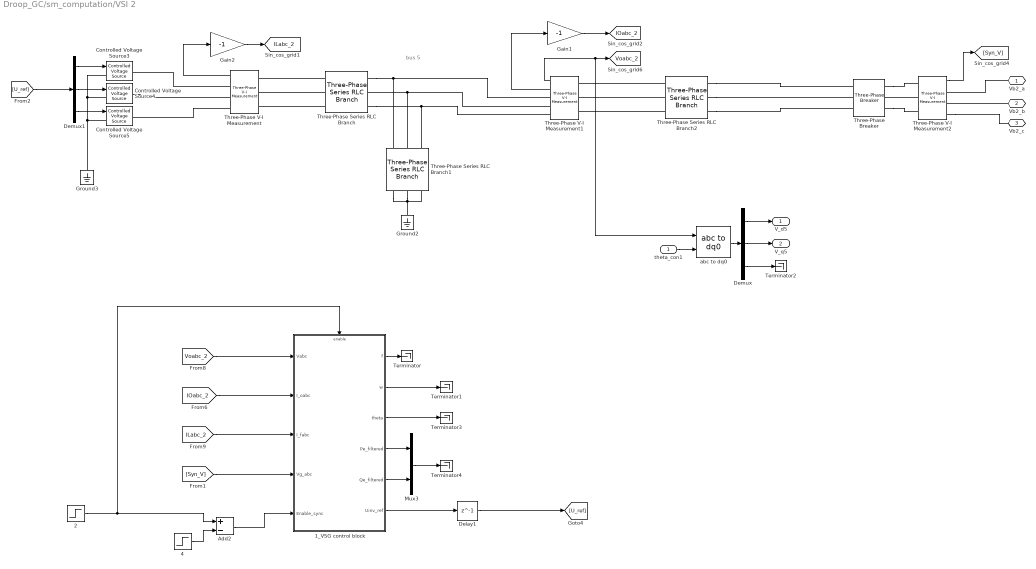
== system Droop_GC/sm_computation/VSI 2 ==
  note: bus 5
  "theta_con1 " : Inport
  " 2" : Step  Time=t_preSyn_start_2  SampleTime=0
  " 4" : Step  Time=t_preSyn_end_2  SampleTime=0
  1_VSG control block : Subsystem
  Add2 : Sum  Inputs=+-
  Controlled Voltage Source3 : powerlib/Electrical Sources/Controlled Voltage Source  Initialize=on  Source_Type=AC  Amplitude=0  Phase=0  Frequency=0  Measurements=None
  Controlled Voltage Source4 : powerlib/Electrical Sources/Controlled Voltage Source  Initialize=on  Source_Type=AC  Amplitude=0  Phase=0  Frequency=0  Measurements=None
  Controlled Voltage Source5 : powerlib/Electrical Sources/Controlled Voltage Source  Initialize=on  Source_Type=AC  Amplitude=0  Phase=0  Frequency=0  Measurements=None
  Delay1 : Delay  DelayLength=1  InitialCondition=0
  Demux : Demux  Outputs=3
  Demux1 : Demux  Outputs=3
  Gain1 : Gain  Gain=-1
  Gain2 : Gain  Gain=-1
  Ground2 : powerlib/Elements/Ground  LConnTagsString=a
  Ground3 : powerlib/Elements/Ground  LConnTagsString=a
  Mux3 : Mux  Inputs=2
  Terminator{,1..4} (5 alike) : Terminator
  Three-Phase Series RLC Branch : powerlib/Elements/Three-Phase Series RLC Branch  LConnTagsString=A|B|C  RConnTagsString=A|B|C  BranchType=RL  Resistance=Rf_2  Inductance=Lf_2  Capacitance=1e-6  Measurements=None
  Three-Phase Series RLC Branch1 : powerlib/Elements/Three-Phase Series RLC Branch  LConnTagsString=A|B|C  RConnTagsString=A|B|C  BranchType=C  Resistance=Rf_1  Inductance=0.1e-3  Capacitance=Cf_2  Measurements=None
  Three-Phase Series RLC Branch2 : powerlib/Elements/Three-Phase Series RLC Branch  LConnTagsString=A|B|C  RConnTagsString=A|B|C  BranchType=RL  Resistance=R_2  Inductance=L_2  Capacitance=1e-6  Measurements=None
  Three-Phase V-I Measurement : powerlib/Measurements/Three-Phase V-I Measurement  VoltageMeasurement=no  SetLabelV=off  LabelV=Vabc  Vpu=off  VpuLL=off  CurrentMeasurement=yes  SetLabelI=off  LabelI=Iabc  Ipu=off  Pbase=100e6  Vbase=500e3  OutputType=Complex  PhasorSimulation=off  PSBequivalent=0
  Three-Phase V-I Measurement1 : powerlib/Measurements/Three-Phase V-I Measurement  VoltageMeasurement=phase-to-ground  SetLabelV=off  LabelV=Vabc  Vpu=off  VpuLL=off  CurrentMeasurement=yes  SetLabelI=off  LabelI=Iabc  Ipu=off  Pbase=100e6  Vbase=500e3  OutputType=Complex  PhasorSimulation=off  PSBequivalent=0
  Three-Phase V-I Measurement2 : powerlib/Measurements/Three-Phase V-I Measurement  VoltageMeasurement=phase-to-ground  SetLabelV=off  LabelV=Vabc  Vpu=off  VpuLL=off  CurrentMeasurement=no  SetLabelI=off  LabelI=Iabc  Ipu=off  Pbase=100e6  Vbase=500e3  OutputType=Complex  PhasorSimulation=off  PSBequivalent=0
  Three-Phase Breaker : powerlib/Elements/Three-Phase Breaker  InitialState=open  SwitchA=on  SwitchB=on  SwitchC=on  SwitchTimes="[t_grid_breaker_2  20]"  External=off  BreakerResistance=0.00001  SnubberResistance=1e8  SnubberCapacitance=inf  Measurements=None
  abc to dq0 : powerlib_meascontrol/Transformations/abc to dq0  Alignment=Aligned with phase A axis
  Vb2_a : PMIOPort  Side=Right
  Vb2_b : PMIOPort  Port=2  Side=Right
  Vb2_c : PMIOPort  Port=3  Side=Right
  V_d5 : Outport
  V_q5 : Outport  Port=2
  tag scope: ILabc_2=global, IOabc_2=global, Voabc_2=global
  wires:
  1_VSG control block/3(theta) -> Terminator3/1
  [IOabc_2] -> 1_VSG control block/2(I_oabc)
  [Voabc_2] -> 1_VSG control block/1(Vabc)
  [ILabc_2] -> 1_VSG control block/3(I_fabc)
  Mux3/1 -> Terminator4/1
  1_VSG control block/4(Pe_filtered) -> Mux3/1
  1_VSG control block/5(Qe_filtered) -> Mux3/2
  1_VSG control block/2(w) -> Terminator1/1
  1_VSG control block/1(f) -> Terminator/1
  Three-Phase V-I Measurement2/1 -> [Syn_V]
  [Syn_V] -> 1_VSG control block/4(Vg_abc)
  " 4"/1 -> Add2/2
  " 2"/1 -> Add2/1, 1_VSG control block/Enable
  Add2/1 -> 1_VSG control block/5(Enable_sync)
  Three-Phase V-I Measurement1/2 -> Gain1/1
  Gain2/1 -> [ILabc_2]
  Three-Phase V-I Measurement/1 -> Gain2/1
  Gain1/1 -> [IOabc_2]
  Delay1/1 -> [U_ref]
  1_VSG control block/6(Uinv_ref) -> Delay1/1
  Demux/2 -> V_q5/1
  Demux/3 -> Terminator2/1
  Demux/1 -> V_d5/1
  abc to dq0/1 -> Demux/1
  "theta_con1 "/1 -> abc to dq0/2
  Three-Phase V-I Measurement1/1 -> abc to dq0/1, [Voabc_2]
  Demux1/1 -> Controlled Voltage Source3/1
  Demux1/3 -> Controlled Voltage Source5/1
  Demux1/2 -> Controlled Voltage Source4/1
  [U_ref] -> Demux1/1
  connections:
  Three-Phase Series RLC Branch2/RConn2 -- Three-Phase Breaker/LConn2
  Three-Phase Series RLC Branch2/RConn3 -- Three-Phase Breaker/LConn3
  Three-Phase Series RLC Branch2/RConn1 -- Three-Phase Breaker/LConn1
  Vb2_b/RConn1 -- Three-Phase V-I Measurement2/RConn2
  Three-Phase Breaker/RConn3 -- Three-Phase V-I Measurement2/LConn3
  Vb2_a/RConn1 -- Three-Phase V-I Measurement2/RConn1
  Three-Phase V-I Measurement2/RConn3 -- Vb2_c/RConn1
  Three-Phase V-I Measurement2/LConn2 -- Three-Phase Breaker/RConn2
  Three-Phase Breaker/RConn1 -- Three-Phase V-I Measurement2/LConn1
  Three-Phase Series RLC Branch1/RConn1 -- Ground2/LConn1 -- Three-Phase Series RLC Branch1/RConn3 -- Three-Phase Series RLC Branch1/RConn2
  Three-Phase Series RLC Branch2/LConn2 -- Three-Phase V-I Measurement1/LConn2
  Three-Phase Series RLC Branch/LConn2 -- Three-Phase V-I Measurement/LConn2
  Three-Phase Series RLC Branch/LConn1 -- Three-Phase V-I Measurement/LConn1
  Three-Phase Series RLC Branch2/LConn3 -- Three-Phase V-I Measurement1/LConn3
  Three-Phase Series RLC Branch/LConn3 -- Three-Phase V-I Measurement/LConn3
  Three-Phase Series RLC Branch2/LConn1 -- Three-Phase V-I Measurement1/LConn1
  Three-Phase Series RLC Branch/RConn1 -- Three-Phase Series RLC Branch1/LConn1 -- Three-Phase V-I Measurement1/RConn1
  Three-Phase V-I Measurement1/RConn2 -- Three-Phase Series RLC Branch/RConn2 -- Three-Phase Series RLC Branch1/LConn2
  Three-Phase Series RLC Branch/RConn3 -- Three-Phase Series RLC Branch1/LConn3 -- Three-Phase V-I Measurement1/RConn3
  Controlled Voltage Source3/LConn1 -- Controlled Voltage Source4/LConn1 -- Ground3/LConn1 -- Controlled Voltage Source5/LConn1
  Three-Phase V-I Measurement/RConn2 -- Controlled Voltage Source4/RConn1
  Three-Phase V-I Measurement/RConn1 -- Controlled Voltage Source3/RConn1
  Three-Phase V-I Measurement/RConn3 -- Controlled Voltage Source5/RConn1

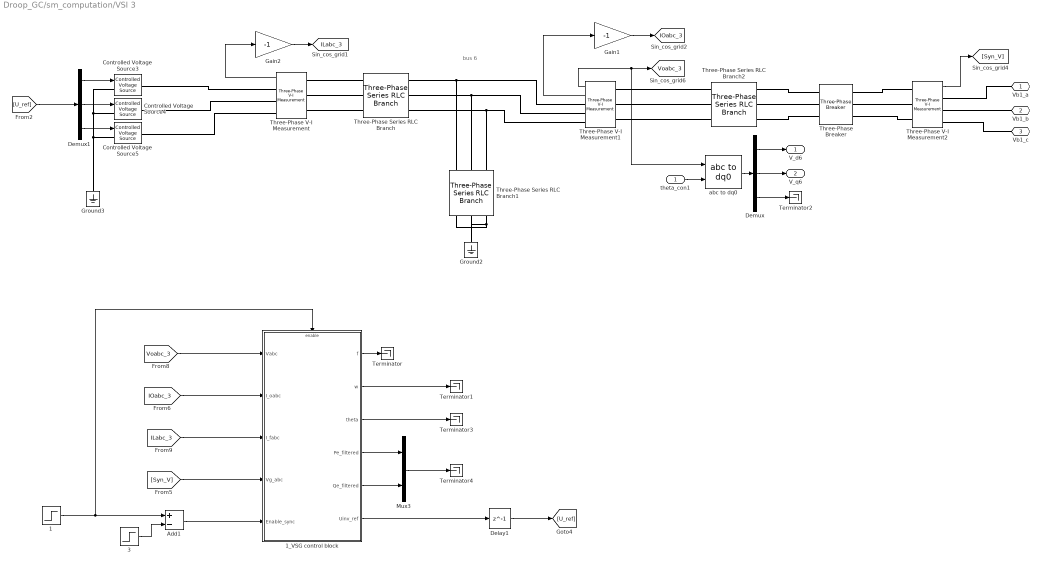
== system Droop_GC/sm_computation/VSI 3 ==
  note: bus 6
  "theta_con1 " : Inport
  " 1" : Step  Time=t_preSyn_start_3  SampleTime=0
  " 3" : Step  Time=t_preSyn_end_3  SampleTime=0
  1_VSG control block : Subsystem
  Add1 : Sum  Inputs=+-
  Controlled Voltage Source3 : powerlib/Electrical Sources/Controlled Voltage Source  Initialize=on  Source_Type=AC  Amplitude=0  Phase=0  Frequency=0  Measurements=None
  Controlled Voltage Source4 : powerlib/Electrical Sources/Controlled Voltage Source  Initialize=on  Source_Type=AC  Amplitude=0  Phase=0  Frequency=0  Measurements=None
  Controlled Voltage Source5 : powerlib/Electrical Sources/Controlled Voltage Source  Initialize=on  Source_Type=AC  Amplitude=0  Phase=0  Frequency=0  Measurements=None
  Delay1 : Delay  DelayLength=1  InitialCondition=0
  Demux : Demux  Outputs=3
  Demux1 : Demux  Outputs=3
  Gain1 : Gain  Gain=-1
  Gain2 : Gain  Gain=-1
  Ground2 : powerlib/Elements/Ground  LConnTagsString=a
  Ground3 : powerlib/Elements/Ground  LConnTagsString=a
  Mux3 : Mux  Inputs=2
  Terminator{,1..4} (5 alike) : Terminator
  Three-Phase Series RLC Branch : powerlib/Elements/Three-Phase Series RLC Branch  LConnTagsString=A|B|C  RConnTagsString=A|B|C  BranchType=RL  Resistance=Rf_3  Inductance=Lf_3  Capacitance=1e-6  Measurements=None
  Three-Phase Series RLC Branch1 : powerlib/Elements/Three-Phase Series RLC Branch  LConnTagsString=A|B|C  RConnTagsString=A|B|C  BranchType=C  Resistance=Rf_1  Inductance=0.1e-3  Capacitance=Cf_3  Measurements=None
  Three-Phase Series RLC Branch2 : powerlib/Elements/Three-Phase Series RLC Branch  LConnTagsString=A|B|C  RConnTagsString=A|B|C  BranchType=RL  Resistance=R_3  Inductance=L_3  Capacitance=1e-6  Measurements=None
  Three-Phase V-I Measurement : powerlib/Measurements/Three-Phase V-I Measurement  VoltageMeasurement=no  SetLabelV=off  LabelV=Vabc  Vpu=off  VpuLL=off  CurrentMeasurement=yes  SetLabelI=off  LabelI=Iabc  Ipu=off  Pbase=100e6  Vbase=500e3  OutputType=Complex  PhasorSimulation=off  PSBequivalent=0
  Three-Phase V-I Measurement1 : powerlib/Measurements/Three-Phase V-I Measurement  VoltageMeasurement=phase-to-ground  SetLabelV=off  LabelV=Vabc  Vpu=off  VpuLL=off  CurrentMeasurement=yes  SetLabelI=off  LabelI=Iabc  Ipu=off  Pbase=100e6  Vbase=500e3  OutputType=Complex  PhasorSimulation=off  PSBequivalent=0
  Three-Phase V-I Measurement2 : powerlib/Measurements/Three-Phase V-I Measurement  VoltageMeasurement=phase-to-ground  SetLabelV=off  LabelV=Vabc  Vpu=off  VpuLL=off  CurrentMeasurement=no  SetLabelI=off  LabelI=Iabc  Ipu=off  Pbase=100e6  Vbase=500e3  OutputType=Complex  PhasorSimulation=off  PSBequivalent=0
  Three-Phase Breaker : powerlib/Elements/Three-Phase Breaker  InitialState=open  SwitchA=on  SwitchB=on  SwitchC=on  SwitchTimes="[t_grid_breaker_3  20]"  External=off  BreakerResistance=0.00001  SnubberResistance=1e8  SnubberCapacitance=inf  Measurements=None
  abc to dq0 : powerlib_meascontrol/Transformations/abc to dq0  Alignment=Aligned with phase A axis
  Vb1_a : PMIOPort  Side=Right
  Vb1_b : PMIOPort  Port=2  Side=Right
  Vb1_c : PMIOPort  Port=3  Side=Right
  V_d6 : Outport
  V_q6 : Outport  Port=2
  tag scope: ILabc_3=global, IOabc_3=global, Voabc_3=global
  wires:
  [ILabc_3] -> 1_VSG control block/3(I_fabc)
  [Voabc_3] -> 1_VSG control block/1(Vabc)
  [IOabc_3] -> 1_VSG control block/2(I_oabc)
  1_VSG control block/3(theta) -> Terminator3/1
  Mux3/1 -> Terminator4/1
  1_VSG control block/4(Pe_filtered) -> Mux3/1
  1_VSG control block/5(Qe_filtered) -> Mux3/2
  1_VSG control block/2(w) -> Terminator1/1
  1_VSG control block/1(f) -> Terminator/1
  Three-Phase V-I Measurement2/1 -> [Syn_V]
  [Syn_V] -> 1_VSG control block/4(Vg_abc)
  " 3"/1 -> Add1/2
  " 1"/1 -> 1_VSG control block/Enable, Add1/1
  Add1/1 -> 1_VSG control block/5(Enable_sync)
  Three-Phase V-I Measurement1/1 -> abc to dq0/1, [Voabc_3]
  Gain1/1 -> [IOabc_3]
  Three-Phase V-I Measurement/1 -> Gain2/1
  Three-Phase V-I Measurement1/2 -> Gain1/1
  Gain2/1 -> [ILabc_3]
  Delay1/1 -> [U_ref]
  1_VSG control block/6(Uinv_ref) -> Delay1/1
  "theta_con1 "/1 -> abc to dq0/2
  Demux/2 -> V_q6/1
  Demux/1 -> V_d6/1
  abc to dq0/1 -> Demux/1
  Demux/3 -> Terminator2/1
  Demux1/2 -> Controlled Voltage Source4/1
  [U_ref] -> Demux1/1
  Demux1/3 -> Controlled Voltage Source5/1
  Demux1/1 -> Controlled Voltage Source3/1
  connections:
  Three-Phase Series RLC Branch2/RConn3 -- Three-Phase Breaker/LConn3
  Three-Phase Series RLC Branch2/RConn2 -- Three-Phase Breaker/LConn2
  Three-Phase Series RLC Branch2/RConn1 -- Three-Phase Breaker/LConn1
  Vb1_a/RConn1 -- Three-Phase V-I Measurement2/RConn1
  Three-Phase Breaker/RConn3 -- Three-Phase V-I Measurement2/LConn3
  Vb1_b/RConn1 -- Three-Phase V-I Measurement2/RConn2
  Three-Phase V-I Measurement2/LConn2 -- Three-Phase Breaker/RConn2
  Vb1_c/RConn1 -- Three-Phase V-I Measurement2/RConn3
  Three-Phase Breaker/RConn1 -- Three-Phase V-I Measurement2/LConn1
  Three-Phase Series RLC Branch1/RConn3 -- Three-Phase Series RLC Branch1/RConn1 -- Three-Phase Series RLC Branch1/RConn2 -- Ground2/LConn1
  Three-Phase V-I Measurement/LConn3 -- Three-Phase Series RLC Branch/LConn3
  Three-Phase V-I Measurement/LConn1 -- Three-Phase Series RLC Branch/LConn1
  Three-Phase V-I Measurement/LConn2 -- Three-Phase Series RLC Branch/LConn2
  Three-Phase Series RLC Branch2/LConn1 -- Three-Phase V-I Measurement1/LConn1
  Three-Phase Series RLC Branch2/LConn3 -- Three-Phase V-I Measurement1/LConn3
  Three-Phase Series RLC Branch2/LConn2 -- Three-Phase V-I Measurement1/LConn2
  Three-Phase Series RLC Branch/RConn1 -- Three-Phase Series RLC Branch1/LConn1 -- Three-Phase V-I Measurement1/RConn1
  Three-Phase V-I Measurement1/RConn2 -- Three-Phase Series RLC Branch1/LConn2 -- Three-Phase Series RLC Branch/RConn2
  Three-Phase Series RLC Branch/RConn3 -- Three-Phase Series RLC Branch1/LConn3 -- Three-Phase V-I Measurement1/RConn3
  Controlled Voltage Source4/LConn1 -- Ground3/LConn1 -- Controlled Voltage Source5/LConn1 -- Controlled Voltage Source3/LConn1
  Three-Phase V-I Measurement/RConn3 -- Controlled Voltage Source5/RConn1
  Three-Phase V-I Measurement/RConn1 -- Controlled Voltage Source3/RConn1
  Three-Phase V-I Measurement/RConn2 -- Controlled Voltage Source4/RConn1

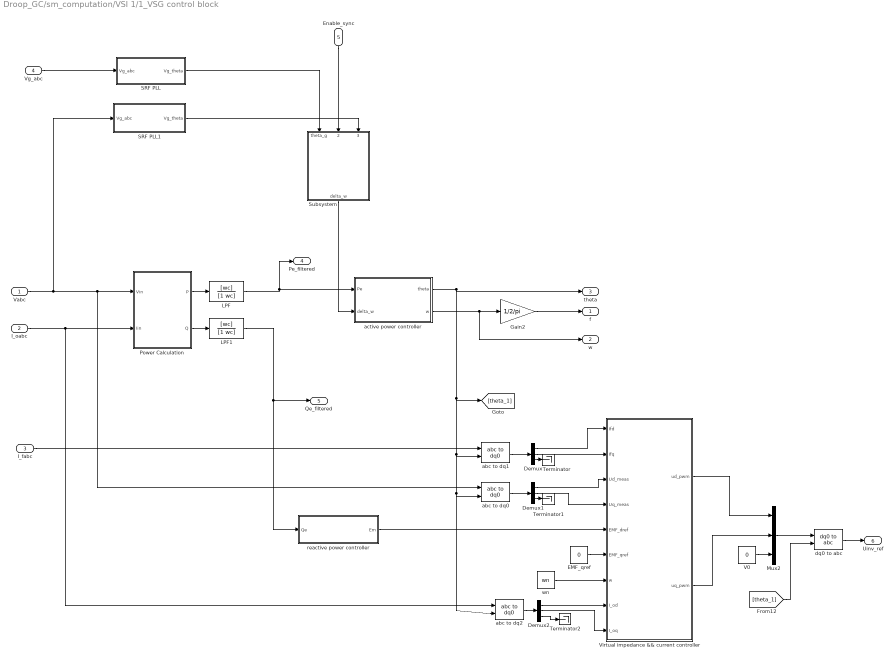
== system Droop_GC/sm_computation/VSI 1/1_VSG control block ==
  Vabc : Inport
  I_oabc : Inport  Port=2
  I_fabc : Inport  Port=3
  Vg_abc : Inport  Port=4
  Enable_sync : Inport  Port=5
  Demux : Demux  Outputs=3
  Demux1 : Demux  Outputs=3
  Demux2 : Demux  Outputs=3
  EMF_qref : Constant  Value=0
  Gain2 : Gain  Gain=1/2/pi
  LPF : TransferFcn  Numerator=[wc]  Denominator=[1 wc]
  LPF1 : TransferFcn  Numerator=[wc]  Denominator=[1 wc]
  Mux2 : Mux  Inputs=3
  Power Calculation : Subsystem
  SRF PLL : Subsystem
  SRF PLL1 : Subsystem
  Subsystem : Subsystem
  Terminator : Terminator
  Terminator1 : Terminator
  Terminator2 : Terminator
  V0 : Constant  Value=0
  Virtual impedance && current controller : Subsystem
  abc to dq0 : powerlib_meascontrol/Transformations/abc to dq0  Alignment=Aligned with phase A axis
  abc to dq1 : powerlib_meascontrol/Transformations/abc to dq0  Alignment=Aligned with phase A axis
  abc to dq2 : powerlib_meascontrol/Transformations/abc to dq0  Alignment=Aligned with phase A axis
  active power controller : Subsystem
  dq0 to abc : powerlib_meascontrol/Transformations/dq0 to abc  Alignment=Aligned with phase A axis
  reactive power controller : Subsystem
  wn : Constant  Value=wn
  f : Outport
  w : Outport  Port=2
  theta : Outport  Port=3
  Pe_filtered : Outport  Port=4
  Qe_filtered : Outport  Port=5
  Uinv_ref : Outport  Port=6
  wires:
  Demux1/2 -> Virtual impedance && current controller/4(Uq_meas)
  dq0 to abc/1 -> Uinv_ref/1
  Demux1/1 -> Virtual impedance && current controller/3(Ud_meas)
  Demux/1 -> Virtual impedance && current controller/1(Ifd)
  abc to dq1/1 -> Demux/1
  Demux/2 -> Virtual impedance && current controller/2(Ifq)
  V0/1 -> Mux2/3
  [theta_1] -> dq0 to abc/2
  Mux2/1 -> dq0 to abc/1
  abc to dq0/1 -> Demux1/1
  I_oabc/1 -> Power Calculation/2(Iin), abc to dq2/1
  Gain2/1 -> f/1
  Power Calculation/1(P) -> LPF/1
  Power Calculation/2(Q) -> LPF1/1
  active power controller/1(theta) -> theta/1, abc to dq0/2, abc to dq2/2, abc to dq1/2, [theta_1]
  EMF_qref/1 -> Virtual impedance && current controller/6(EMF_qref)
  Virtual impedance && current controller/2(uq_pwm) -> Mux2/2
  Virtual impedance && current controller/1(ud_pwm) -> Mux2/1
  I_fabc/1 -> abc to dq1/1
  abc to dq2/1 -> Demux2/1
  Demux2/1 -> Virtual impedance && current controller/8(I_od)
  Demux2/2 -> Virtual impedance && current controller/9(I_oq)
  Demux/3 -> Terminator/1
  Demux1/3 -> Terminator1/1
  Demux2/3 -> Terminator2/1
  wn/1 -> Virtual impedance && current controller/7(w)
  reactive power controller/1(Em) -> Virtual impedance && current controller/5(EMF_dref)
  LPF/1 -> active power controller/1(Pe), Pe_filtered/1
  LPF1/1 -> Qe_filtered/1, reactive power controller/1(Qe)
  active power controller/2(w) -> w/1, Gain2/1
  Enable_sync/1 -> Subsystem/2(Enable_sync)
  Vabc/1 -> SRF PLL1/1(Vg_abc), Power Calculation/1(Vin), abc to dq0/1
  SRF PLL/1(Vg_theta) -> Subsystem/1(theta_g)
  Vg_abc/1 -> SRF PLL/1(Vg_abc)
  SRF PLL1/1(Vg_theta) -> Subsystem/3(theta_vsg)
  Subsystem/1(delta_w) -> active power controller/2(delta_w)

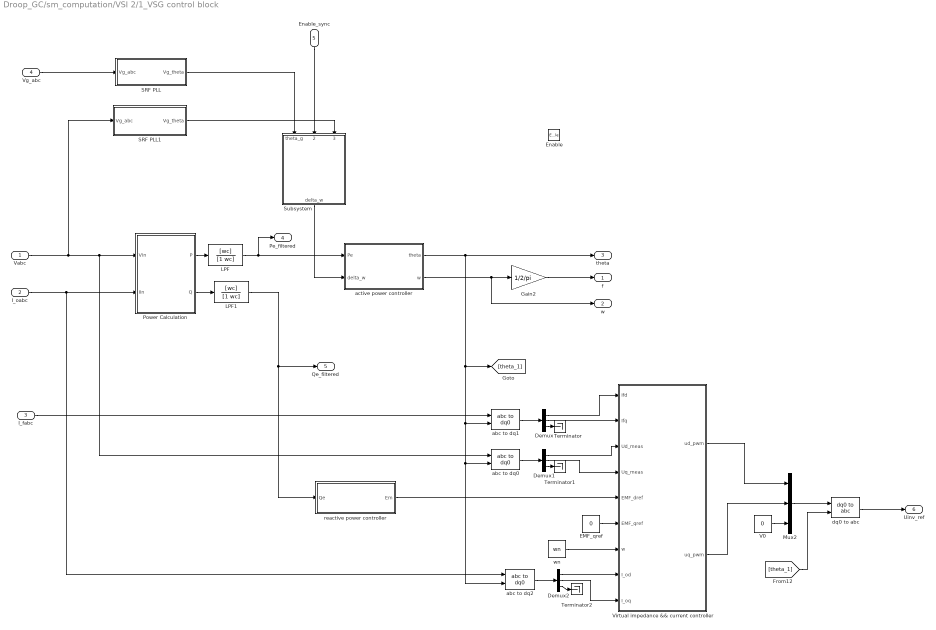
== system Droop_GC/sm_computation/VSI 2/1_VSG control block ==
  Vabc : Inport
  I_oabc : Inport  Port=2
  I_fabc : Inport  Port=3
  Vg_abc : Inport  Port=4
  Enable_sync : Inport  Port=5
  Enable : EnablePort
  Demux : Demux  Outputs=3
  Demux1 : Demux  Outputs=3
  Demux2 : Demux  Outputs=3
  EMF_qref : Constant  Value=0
  Gain2 : Gain  Gain=1/2/pi
  LPF : TransferFcn  Numerator=[wc]  Denominator=[1 wc]
  LPF1 : TransferFcn  Numerator=[wc]  Denominator=[1 wc]
  Mux2 : Mux  Inputs=3
  Power Calculation : Subsystem
  SRF PLL : Subsystem
  SRF PLL1 : Subsystem
  Subsystem : Subsystem
  Terminator : Terminator
  Terminator1 : Terminator
  Terminator2 : Terminator
  V0 : Constant  Value=0
  Virtual impedance && current controller : Subsystem
  abc to dq0 : powerlib_meascontrol/Transformations/abc to dq0  Alignment=Aligned with phase A axis
  abc to dq1 : powerlib_meascontrol/Transformations/abc to dq0  Alignment=Aligned with phase A axis
  abc to dq2 : powerlib_meascontrol/Transformations/abc to dq0  Alignment=Aligned with phase A axis
  active power controller : Subsystem
  dq0 to abc : powerlib_meascontrol/Transformations/dq0 to abc  Alignment=Aligned with phase A axis
  reactive power controller : Subsystem
  wn : Constant  Value=wn
  f : Outport
  w : Outport  Port=2
  theta : Outport  Port=3
  Pe_filtered : Outport  Port=4
  Qe_filtered : Outport  Port=5
  Uinv_ref : Outport  Port=6
  wires:
  LPF1/1 -> reactive power controller/1(Qe), Qe_filtered/1
  LPF/1 -> active power controller/1(Pe), Pe_filtered/1
  reactive power controller/1(Em) -> Virtual impedance && current controller/5(EMF_dref)
  wn/1 -> Virtual impedance && current controller/7(w)
  Demux2/3 -> Terminator2/1
  Demux1/3 -> Terminator1/1
  Demux/3 -> Terminator/1
  Demux2/2 -> Virtual impedance && current controller/9(I_oq)
  Demux2/1 -> Virtual impedance && current controller/8(I_od)
  abc to dq2/1 -> Demux2/1
  I_fabc/1 -> abc to dq1/1
  Virtual impedance && current controller/1(ud_pwm) -> Mux2/1
  Virtual impedance && current controller/2(uq_pwm) -> Mux2/2
  EMF_qref/1 -> Virtual impedance && current controller/6(EMF_qref)
  active power controller/1(theta) -> [theta_1], abc to dq1/2, abc to dq2/2, abc to dq0/2, theta/1
  Power Calculation/2(Q) -> LPF1/1
  Power Calculation/1(P) -> LPF/1
  Gain2/1 -> f/1
  I_oabc/1 -> Power Calculation/2(Iin), abc to dq2/1
  active power controller/2(w) -> Gain2/1, w/1
  abc to dq0/1 -> Demux1/1
  Mux2/1 -> dq0 to abc/1
  [theta_1] -> dq0 to abc/2
  V0/1 -> Mux2/3
  Demux/2 -> Virtual impedance && current controller/2(Ifq)
  abc to dq1/1 -> Demux/1
  Demux/1 -> Virtual impedance && current controller/1(Ifd)
  Demux1/1 -> Virtual impedance && current controller/3(Ud_meas)
  dq0 to abc/1 -> Uinv_ref/1
  Demux1/2 -> Virtual impedance && current controller/4(Uq_meas)
  SRF PLL/1(Vg_theta) -> Subsystem/1(theta_g)
  Vabc/1 -> SRF PLL1/1(Vg_abc), Power Calculation/1(Vin), abc to dq0/1
  Enable_sync/1 -> Subsystem/2(Enable_sync)
  Vg_abc/1 -> SRF PLL/1(Vg_abc)
  SRF PLL1/1(Vg_theta) -> Subsystem/3(theta_vsg)
  Subsystem/1(delta_w) -> active power controller/2(delta_w)

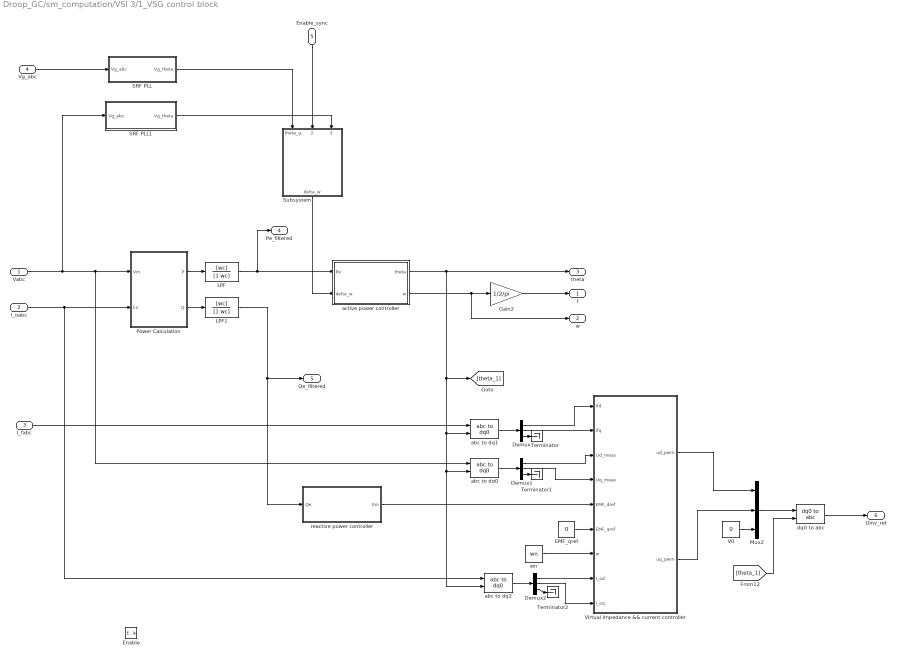
== system Droop_GC/sm_computation/VSI 3/1_VSG control block ==
  Vabc : Inport
  I_oabc : Inport  Port=2
  I_fabc : Inport  Port=3
  Vg_abc : Inport  Port=4
  Enable_sync : Inport  Port=5
  Enable : EnablePort
  Demux : Demux  Outputs=3
  Demux1 : Demux  Outputs=3
  Demux2 : Demux  Outputs=3
  EMF_qref : Constant  Value=0
  Gain2 : Gain  Gain=1/2/pi
  LPF : TransferFcn  Numerator=[wc]  Denominator=[1 wc]
  LPF1 : TransferFcn  Numerator=[wc]  Denominator=[1 wc]
  Mux2 : Mux  Inputs=3
  Power Calculation : Subsystem
  SRF PLL : Subsystem
  SRF PLL1 : Subsystem
  Subsystem : Subsystem
  Terminator : Terminator
  Terminator1 : Terminator
  Terminator2 : Terminator
  V0 : Constant  Value=0
  Virtual impedance && current controller : Subsystem
  abc to dq0 : powerlib_meascontrol/Transformations/abc to dq0  Alignment=Aligned with phase A axis
  abc to dq1 : powerlib_meascontrol/Transformations/abc to dq0  Alignment=Aligned with phase A axis
  abc to dq2 : powerlib_meascontrol/Transformations/abc to dq0  Alignment=Aligned with phase A axis
  active power controller : Subsystem
  dq0 to abc : powerlib_meascontrol/Transformations/dq0 to abc  Alignment=Aligned with phase A axis
  reactive power controller : Subsystem
  wn : Constant  Value=wn
  f : Outport
  w : Outport  Port=2
  theta : Outport  Port=3
  Pe_filtered : Outport  Port=4
  Qe_filtered : Outport  Port=5
  Uinv_ref : Outport  Port=6
  wires:
  Demux1/2 -> Virtual impedance && current controller/4(Uq_meas)
  dq0 to abc/1 -> Uinv_ref/1
  Demux1/1 -> Virtual impedance && current controller/3(Ud_meas)
  Demux/1 -> Virtual impedance && current controller/1(Ifd)
  abc to dq1/1 -> Demux/1
  Demux/2 -> Virtual impedance && current controller/2(Ifq)
  V0/1 -> Mux2/3
  [theta_1] -> dq0 to abc/2
  Mux2/1 -> dq0 to abc/1
  abc to dq0/1 -> Demux1/1
  active power controller/2(w) -> w/1, Gain2/1
  I_oabc/1 -> Power Calculation/2(Iin), abc to dq2/1
  Gain2/1 -> f/1
  Power Calculation/1(P) -> LPF/1
  Power Calculation/2(Q) -> LPF1/1
  active power controller/1(theta) -> theta/1, abc to dq0/2, abc to dq2/2, abc to dq1/2, [theta_1]
  EMF_qref/1 -> Virtual impedance && current controller/6(EMF_qref)
  Virtual impedance && current controller/2(uq_pwm) -> Mux2/2
  Virtual impedance && current controller/1(ud_pwm) -> Mux2/1
  I_fabc/1 -> abc to dq1/1
  abc to dq2/1 -> Demux2/1
  Demux2/1 -> Virtual impedance && current controller/8(I_od)
  Demux2/2 -> Virtual impedance && current controller/9(I_oq)
  Demux/3 -> Terminator/1
  Demux1/3 -> Terminator1/1
  Demux2/3 -> Terminator2/1
  wn/1 -> Virtual impedance && current controller/7(w)
  reactive power controller/1(Em) -> Virtual impedance && current controller/5(EMF_dref)
  LPF/1 -> active power controller/1(Pe), Pe_filtered/1
  LPF1/1 -> Qe_filtered/1, reactive power controller/1(Qe)
  SRF PLL1/1(Vg_theta) -> Subsystem/3(theta_vsg)
  Vg_abc/1 -> SRF PLL/1(Vg_abc)
  Enable_sync/1 -> Subsystem/2(Enable_sync)
  Vabc/1 -> SRF PLL1/1(Vg_abc), Power Calculation/1(Vin), abc to dq0/1
  SRF PLL/1(Vg_theta) -> Subsystem/1(theta_g)
  Subsystem/1(delta_w) -> active power controller/2(delta_w)

== system Droop_GC/sm_computation/VSI 1/1_VSG control block/Power Calculation ==
  note: Iabc
  note: Vabc
  Vin : Inport
  Iin : Inport  Port=2
  Add : Sum
  Add1 : Sum  Inputs=-+
  Demux1 : Demux  Outputs=3
  Demux2 : Demux  Outputs=3
  Gain1 : Gain  Gain=3/2
  Gain2 : Gain  Gain=3/2
  Product{,1..3} (4 alike) : Product
  Terminator : Terminator
  Terminator1 : Terminator
  abc to Alpha-Beta-Zero : powerlib_meascontrol/Transformations/abc to Alpha-Beta-Zero
      settings: SourceProductName=Simscape Power Systems
  abc to Alpha-Beta-Zero1 : powerlib_meascontrol/Transformations/abc to Alpha-Beta-Zero
      settings: SourceProductName=Simscape Power Systems
  P : Outport
  Q : Outport  Port=2
  wires:
  Add1/1 -> Gain1/1
  Add/1 -> Gain2/1
  Demux2/2 -> Product1/2, Product2/2
  Product3/1 -> Add1/2
  Product2/1 -> Add1/1
  Product1/1 -> Add/2
  Product/1 -> Add/1
  abc to Alpha-Beta-Zero/1 -> Demux1/1
  Demux1/1 -> Product2/1, Product/1
  abc to Alpha-Beta-Zero1/1 -> Demux2/1
  Demux2/3 -> Terminator1/1
  Demux1/3 -> Terminator/1
  Demux2/1 -> Product3/2, Product/2
  Demux1/2 -> Product3/1, Product1/1
  Vin/1 -> abc to Alpha-Beta-Zero/1
  Iin/1 -> abc to Alpha-Beta-Zero1/1
  Gain2/1 -> P/1
  Gain1/1 -> Q/1

== system Droop_GC/sm_computation/VSI 1/1_VSG control block/SRF PLL ==
  Vg_abc : Inport
  Demux2 : Demux  Outputs=3
  LPF2 : TransferFcn  Numerator=[wf_pll]  Denominator=[1 wf_pll]
  LPF3 : TransferFcn  Numerator=[wf_pll]  Denominator=[1 wf_pll]
  SRF_PLL : Subsystem
  Tclark : Subsystem
  Tpark : Subsystem
  Vg_theta : Outport
  wires:
  Demux2/1 -> Tclark/1(Ua)
  Demux2/2 -> Tclark/2(Ub)
  Demux2/3 -> Tclark/3(Uc)
  Tpark/1(Ud) -> LPF3/1
  Tclark/1(Valpha) -> Tpark/1(Ualpha)
  Tpark/2(Uq) -> LPF2/1
  LPF2/1 -> SRF_PLL/1(vq)  "SRF_vq"
  Vg_abc/1 -> Demux2/1
  Tclark/2(Vbeta) -> Tpark/2(Ubeta)
  SRF_PLL/1(wt) -> Tpark/3(theta), Vg_theta/1  "SRF_wt_mod"
